simulink model "modelo_sistema"  (R2018b)
settings: Solver=VariableStepAuto  StartTime=0.0  StopTime=10.0  RelTol=1e-3
values from neighbouring files (symbols this model uses):
  B = 100    [params.m]
  F = 10    [params.m]
  m = 100    [params.m]
libraries: simulink x1
settings Model: Creator=yasminnunes  LastModifiedBy=yasminnunes

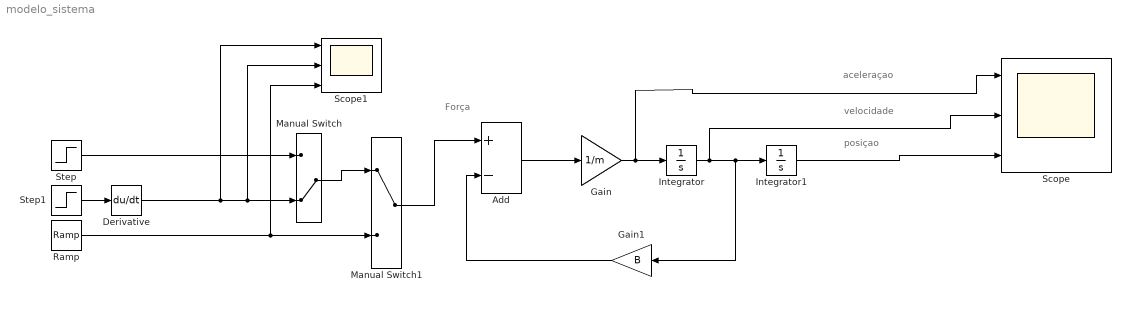
== system modelo_sistema ==
  note: aceleraçao
  note: velocidade
  note: posiçao
  note: Força
  Add : Sum  Inputs=+-
  Derivative : Derivative
  Gain : Gain  Gain=1/m
  Gain1 : Gain  Gain=B
  Integrator : Integrator
  Integrator1 : Integrator
  Manual Switch : ManualSwitch  CurrentSetting=0
  Manual Switch1 : ManualSwitch
  Ramp : simulink/Sources/Ramp  slope=F  start=0  InitialOutput=0
  Scope : Scope  NumInputPorts=3
  Scope1 : Scope  NumInputPorts=3
  Step : Step  After=F  SampleTime=0
  Step1 : Step  After=F  SampleTime=0
  wires:
  Step/1 -> Manual Switch/1
  Add/1 -> Gain/1
  Gain/1 -> Scope/1, Integrator/1
  Integrator/1 -> Scope/2, Gain1/1, Integrator1/1
  Gain1/1 -> Add/2
  Integrator1/1 -> Scope/3
  Manual Switch/1 -> Manual Switch1/1
  Ramp/1 -> Scope1/3, Manual Switch1/2
  Manual Switch1/1 -> Add/1
  Step1/1 -> Derivative/1
  Derivative/1 -> Scope1/1, Scope1/2, Manual Switch/2
